simulink model "mean_spike_rate"  (R2020b)
settings: Solver=FixedStepDiscrete  StartTime=0.0  StopTime=stopTime  FixedStep=2.0833333333333333e-05  RelTol=1e-3
values from neighbouring files (symbols this model uses):
  nSites = 4    [modelparameters.m]
  tabs = 10e-3    (= 0.01)    [modelparameters.m]
  trel = 10e-3    (= 0.01)    [modelparameters.m]
settings Model: Creator=Ross  LastModifiedBy=conno
settings SolverCC: AutoInsertRateTranBlk=on
settings DataIOCC: SaveOutput=off  SaveTime=off  ReturnWorkspaceOutputs=off
settings OptimizationCC: BlockReduction=off  ConditionallyExecuteInputs=off  DefaultParameterBehavior=Inlined
settings DebuggingCC: ReadBeforeWriteMsg=DisableAll  WriteAfterWriteMsg=DisableAll  WriteAfterReadMsg=DisableAll  AlgebraicLoopMsg=error  MultiTaskDSMMsg=none  SingleTaskRateTransMsg=error  PregeneratedLibrarySubsystemCodeDiagnostic=none  ArithmeticOperatorsInVariantConditions=warning
settings HardwareCC: ProdBitPerPointer=32  ProdBitPerSizeT=32  ProdBitPerPtrDiffT=32  ProdLargestAtomicFloat=None  ProdIntDivRoundTo=Undefined  ProdEndianess=Unspecified  ProdWordSize=32  ProdHWDeviceType=ASIC/FPGA->ASIC/FPGA  TargetBitPerPointer=64  TargetBitPerSizeT=64  TargetBitPerPtrDiffT=64  TargetLongLongMode=on  TargetIntDivRoundTo=Zero  TargetEndianess=LittleEndian  TargetWordSize=64  TargetHWDeviceType=Custom Processor->MATLAB Host Computer  ProdEqTarget=off
settings ModelReferenceCC: UpdateModelReferenceTargets=IfOutOfDate
settings SFSimCC: SFSimEcho=off  SimUseLocalCustomCode=off  CustomCodeUndefinedFunction=UseInterfaceOnly
settings RTWCC: RTWUseLocalCustomCode=off

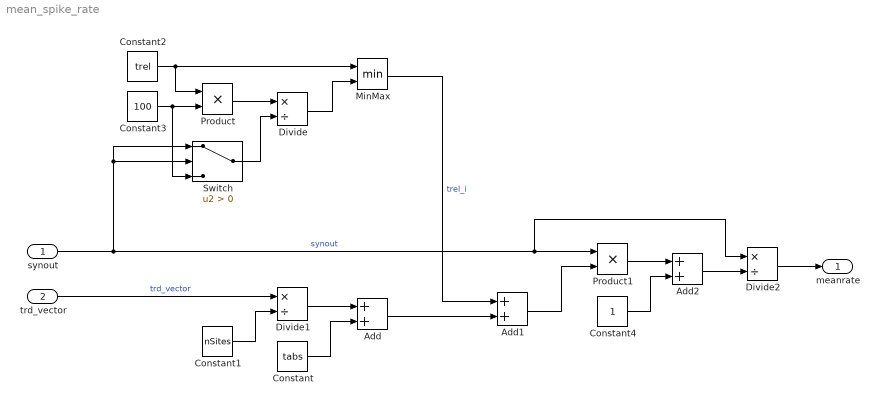
== system mean_spike_rate ==
  synout : Inport  OutDataTypeStr=single  PortDimensions=1  SampleTime=[2.0833333333333333e-05,0]
  trd_vector : Inport  Port=2  OutDataTypeStr=single  PortDimensions=1  SampleTime=[2.0833333333333333e-05,0]
  Add : Sum
  Add1 : Sum
  Add2 : Sum
  Constant : Constant  Value=tabs  OutDataTypeStr=single  SampleTime=-1
  Constant1 : Constant  Value=nSites  OutDataTypeStr=single  SampleTime=-1
  Constant2 : Constant  Value=trel  OutDataTypeStr=single  SampleTime=-1
  Constant3 : Constant  Value=100  OutDataTypeStr=single  SampleTime=-1
  Constant4 : Constant  OutDataTypeStr=single  SampleTime=-1
  Divide : Product  Inputs=*/  RndMeth=Zero  SaturateOnIntegerOverflow=on
  Divide1 : Product  Inputs=*/  RndMeth=Zero  SaturateOnIntegerOverflow=on
  Divide2 : Product  Inputs=*/  RndMeth=Zero  SaturateOnIntegerOverflow=on
  MinMax : MinMax  Inputs=2
  Product : Product
  Product1 : Product
  Switch : Switch  Criteria=u2 > Threshold
  meanrate : Outport  OutDataTypeStr=single  PortDimensions=1  SampleTime=[2.0833333333333333e-05,0]  VectorParamsAs1DForOutWhenUnconnected=off
  wires:
  Switch/1 -> Divide/2
  Divide2/1 -> meanrate/1
  Add2/1 -> Divide2/2
  Product1/1 -> Add2/1
  Add1/1 -> Product1/2
  Constant4/1 -> Add2/2
  Add/1 -> Add1/2
  Constant/1 -> Add/2
  Divide1/1 -> Add/1
  Constant1/1 -> Divide1/2
  MinMax/1 -> Add1/1  "trel_i"
  Divide/1 -> MinMax/2
  Product/1 -> Divide/1
  Constant3/1 -> Switch/3, Product/2
  Constant2/1 -> MinMax/1, Product/1
  trd_vector/1 -> Divide1/1  "trd_vector"
  synout/1 -> Switch/1, Switch/2, Divide2/1, Product1/1  "synout"
